simulink model "stm32_can_telemetry_filter_model"  (R2026a)
settings: Solver=FixedStepDiscrete  StopTime=10  FixedStep=0.01
settings Model: Creator=joshw  LastModifiedBy=joshw

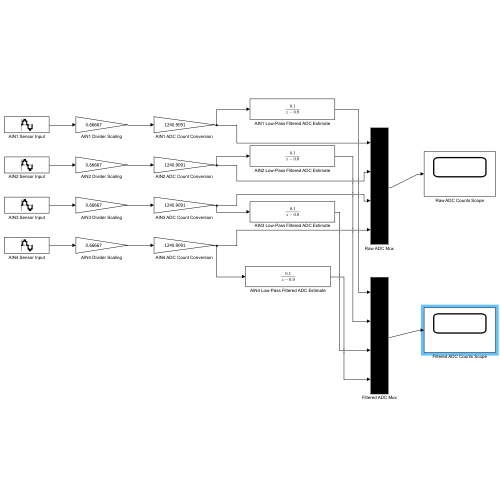
[thumbnail: Simulink's stored preview of the top-level diagram]
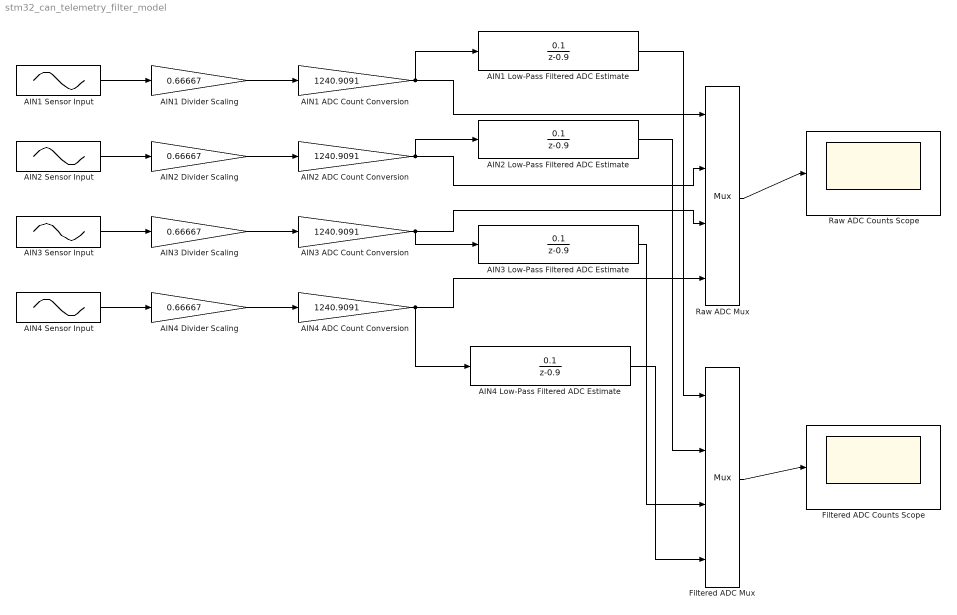
== system stm32_can_telemetry_filter_model ==
  AIN1 ADC Count Conversion : Gain  Gain=1240.9091
  AIN1 Divider Scaling : Gain  Gain=0.66667
  AIN1 Low-Pass Filtered ADC Estimate : DiscreteTransferFcn  Numerator=[0.1]  Denominator=[1 -0.9]  SampleTime=0.01
  AIN1 Sensor Input : Sin  Amplitude=0.4  Bias=1.45  Frequency=0.55  SampleTime=0.01
  AIN2 ADC Count Conversion : Gain  Gain=1240.9091
  AIN2 Divider Scaling : Gain  Gain=0.66667
  AIN2 Low-Pass Filtered ADC Estimate : DiscreteTransferFcn  Numerator=[0.1]  Denominator=[1 -0.9]  SampleTime=0.01
  AIN2 Sensor Input : Sin  Amplitude=0.45  Bias=1.9  Frequency=0.7  SampleTime=0.01
  AIN3 ADC Count Conversion : Gain  Gain=1240.9091
  AIN3 Divider Scaling : Gain  Gain=0.66667
  AIN3 Low-Pass Filtered ADC Estimate : DiscreteTransferFcn  Numerator=[0.1]  Denominator=[1 -0.9]  SampleTime=0.01
  AIN3 Sensor Input : Sin  Amplitude=0.5  Bias=2.35  Frequency=0.85  SampleTime=0.01
  AIN4 ADC Count Conversion : Gain  Gain=1240.9091
  AIN4 Divider Scaling : Gain  Gain=0.66667
  AIN4 Low-Pass Filtered ADC Estimate : DiscreteTransferFcn  Numerator=[0.1]  Denominator=[1 -0.9]  SampleTime=0.01
  AIN4 Sensor Input : Sin  Amplitude=0.55  Bias=2.8  SampleTime=0.01
  Filtered ADC Counts Scope : Scope
      settings: ActiveDisplayYMinimum=-346.16795331161063  ActiveDisplayYMaximum=3115.5115798044963
  Filtered ADC Mux : Mux
  Raw ADC Counts Scope : Scope
      settings: ActiveDisplayYMinimum=630.79886093855316  ActiveDisplayYMaximum=3009.2194256937287
  Raw ADC Mux : Mux
  wires:
  AIN1 Sensor Input/1 -> AIN1 Divider Scaling/1
  AIN1 Divider Scaling/1 -> AIN1 ADC Count Conversion/1
  AIN1 ADC Count Conversion/1 -> AIN1 Low-Pass Filtered ADC Estimate/1, Raw ADC Mux/1
  AIN2 Sensor Input/1 -> AIN2 Divider Scaling/1
  AIN2 Divider Scaling/1 -> AIN2 ADC Count Conversion/1
  AIN2 ADC Count Conversion/1 -> AIN2 Low-Pass Filtered ADC Estimate/1, Raw ADC Mux/2
  AIN3 Sensor Input/1 -> AIN3 Divider Scaling/1
  AIN3 Divider Scaling/1 -> AIN3 ADC Count Conversion/1
  AIN3 ADC Count Conversion/1 -> AIN3 Low-Pass Filtered ADC Estimate/1, Raw ADC Mux/3
  AIN4 Sensor Input/1 -> AIN4 Divider Scaling/1
  AIN4 Divider Scaling/1 -> AIN4 ADC Count Conversion/1
  AIN4 ADC Count Conversion/1 -> AIN4 Low-Pass Filtered ADC Estimate/1, Raw ADC Mux/4
  AIN1 Low-Pass Filtered ADC Estimate/1 -> Filtered ADC Mux/1
  AIN2 Low-Pass Filtered ADC Estimate/1 -> Filtered ADC Mux/2
  AIN3 Low-Pass Filtered ADC Estimate/1 -> Filtered ADC Mux/3
  AIN4 Low-Pass Filtered ADC Estimate/1 -> Filtered ADC Mux/4
  Raw ADC Mux/1 -> Raw ADC Counts Scope/1
  Filtered ADC Mux/1 -> Filtered ADC Counts Scope/1
